simulink model "NHR9410Model96k_2020b"  (R2020b)
settings: Solver=ode45  StartTime=0.0  StopTime=1  FixedStep=0.001  MaxStep=20e-6  RelTol=1e-3
undefined symbols (not defined in the file): Ts
libraries: simulink x85, fl_lib x49, powerlib_meascontrol x27, simulink_extras x24, nesl_utility x13
(part 1 of 4)
settings Model: Creator=opal  LastModifiedBy=mne4
settings DataIOCC: ReturnWorkspaceOutputs=off
settings DebuggingCC: ParameterPrecisionLossMsg=none  ArithmeticOperatorsInVariantConditions=warning
settings SFSimCC: SimUseLocalCustomCode=off  CustomCodeUndefinedFunction=UseInterfaceOnly
settings RTWCC: RTWUseLocalCustomCode=off
settings CodeAppCC: StateflowObjectComments=on
settings SimscapeCC: SimscapeNormalizeSystem=off

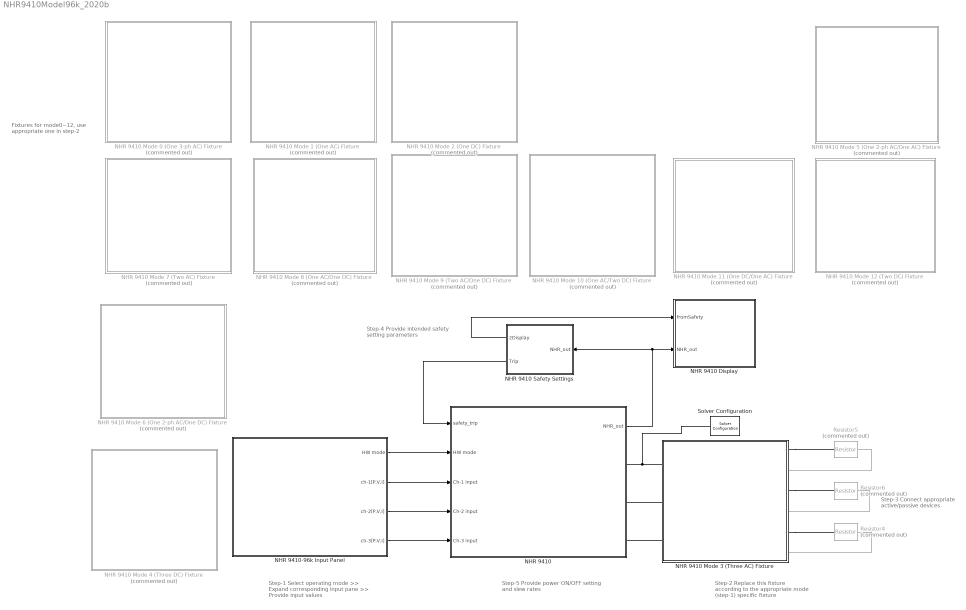
== system NHR9410Model96k_2020b ==
  note: Step-5
      | Provide power ON/OFF setting and slew rates
  note: Step-1
      | Select operating mode >> Expand corresponding input pane >> Provide input values
  note: Step-2
      | Replace this fixture according to the appropriate mode (step-1) specific fixture
  note: Step-3
      | Connect appropriate active/passive devices
  note: Step-4
      | Provide intended safety setting parameters
  note: Fixtures for mode0~12, use appropriate one in step-2
  NHR 9410 : Subsystem  mask{p_switch=1, VslewAC=0.0, FslewAC=500.0, VslewDC=0.0, IslewDC=0.0, PslewDC=0.0}
      mask prompts: p_switch "Enter 1 to turn ON, 0 to turn OFF NHR 9410"
      mask DialogControl DescTextVar Prompt: NHR 9410
      mask DialogControl Container3 Prompt: Slew Rates
      mask DialogControl Control2 Prompt: AC Voltage slew rate [0-500000V/s]:
      mask DialogControl f Prompt: Frequency slew rate [0-500 /s]
      mask DialogControl Control3 Prompt: DC Voltage slew rate [0-20000V/s]:
      mask DialogControl Control4 Prompt: DC current slew rate [0-100000A/s]:
      mask DialogControl Control5 Prompt: DC power slew rate [0-1000000W/s]:
      mask Display: image('NHR9410.png');
  NHR 9410 Display : Subsystem
  NHR 9410 Mode 0 (One 3-ph AC) Fixture : Subsystem  Commented=on
  NHR 9410 Mode 1 (One AC) Fixture : Subsystem  Commented=on
  NHR 9410 Mode 10 (One AC/Two DC) Fixture : Subsystem  Commented=on
  NHR 9410 Mode 11 (One DC/One AC) Fixture : Subsystem  Commented=on
  NHR 9410 Mode 12 (Two DC) Fixture : Subsystem  Commented=on
  NHR 9410 Mode 2 (One DC) Fixture : Subsystem  Commented=on
  NHR 9410 Mode 3 (Three AC) Fixture : Subsystem
  NHR 9410 Mode 4 (Three DC) Fixture : Subsystem  Commented=on
  NHR 9410 Mode 5 (One 2-ph AC/One AC) Fixture : Subsystem  Commented=on
  NHR 9410 Mode 6 (One 2-ph AC/One DC) Fixture : Subsystem  Commented=on
  NHR 9410 Mode 7 (Two AC) Fixture : Subsystem  Commented=on
  NHR 9410 Mode 8 (One AC/One DC) Fixture : Subsystem  Commented=on
  NHR 9410 Mode 9 (Two AC/One DC) Fixture : Subsystem  Commented=on
  NHR 9410 Safety Settings : Subsystem  mask{Vmin1=-50, Tvmin1=2, Svmin1=-1, Vmax1=100, Tvmax1=0.2, Svmax1=-1, Vpeak1=100, Vpeaken1=0, Imaxsrc1=80, Timaxsrc1=2, Simaxsrc1=-1, Imaxsnk1=50, Timaxsnk1=2, Simaxsnk1=-1, Ipeak1=80, Ipeaken1=0, Pmaxsrc1=2000, Tpmaxsrc1=2, Spmaxsrc1=-1, Pmaxsnk1=50, Tpmaxsnk1=2, Spmaxsnk1=-1, Vmin2=-50, Tvmin2=2, Svmin2=-1, Vmax2=90, Tvmax2=0.5, Svmax2=-1, Vpeak2=80, Vpeaken2=0, Imaxsrc2=50, Timaxsrc2=2, Simaxsrc2=-1, Imaxsnk2=8, Timaxsnk2=5, Simaxsnk2=1, Ipeak2=80, Ipeaken2=0, Pmaxsrc2=50, Tpmaxsrc2=2, Spmaxsrc2=-1, Pmaxsnk2=50, Tpmaxsnk2=2, Spmaxsnk2=-1, Vmin3=-50, Tvmin3=2, Svmin3=-1, Vmax3=500, Tvmax3=0.5, Svmax3=-1, Vpeak3=80, Vpeaken3=0, Imaxsrc3=50, Timaxsrc3=2, Simaxsrc3=-1, Imaxsnk3=8, Timaxsnk3=0.2, Simaxsnk3=-1, Ipeak3=80, Ipeaken3=0, Pmaxsrc3=50, Tpmaxsrc3=2, Spmaxsrc3=-1, Pmaxsnk3=3000, Tpmaxsnk3=0.2, Spmaxsnk3=1}
      mask prompts: Vmin1 "Min Voltage (V):"; Tvmin1 "Min Voltage time (S):"; Svmin1 "Enter (-1) to disable safety, 1 to enable:"; Vmax1 "Max Voltage (V):"; Tvmax1 "Max Voltage time (S):"; Svmax1 "Enter (-1) to disable safety, 1 to enable:"; Vpeak1 "Absolute Peak Voltage (V):"; Vpeaken1 "Enable Peak V Trip, yes/no (1/0):"; Imaxsrc1 "Max Source Current (A):"; Timaxsrc1 "Max Source Current Time (S):"; Simaxsrc1 "Enter (-1) to disable safety, 1 to enable:"; Imaxsnk1 "Max Sink Current (A):"; Timaxsnk1 "Max Sink Current Time (S):"; Simaxsnk1 "Enter (-1) to disable safety, 1 to enable:"; Ipeak1 "Absolute Peak Current (A):"; Ipeaken1 "Enable Peak A Trip, yes/no (1/0):"; Pmaxsrc1 "Max Source Power (W):"; Tpmaxsrc1 "Max Source Power Time (S):"; Spmaxsrc1 "Enter (-1) to disable safety, 1 to enable:"; Pmaxsnk1 "Max Sink Power (W):"; Tpmaxsnk1 "Max Sink Power Time (S):"; Spmaxsnk1 "Enter (-1) to disable safety, 1 to enable:"; Vmin2 "Min Voltage (V):"; Tvmin2 "Min Voltage time (S):"; Svmin2 "Enter (-1) to disable safety, 1 to enable:"; Vmax2 "Max Voltage (V):"; Tvmax2 "Max Voltage time (S):"; Svmax2 "Enter (-1) to disable safety, 1 to enable:"; Vpeak2 "Absolute Peak Voltage (V):"; Vpeaken2 "Enable Peak V Trip, yes/no (1/0):"; Imaxsrc2 "Max Source Current (A):"; Timaxsrc2 "Max Source Current Time (S):"; Simaxsrc2 "Enter (-1) to disable safety, 1 to enable:"; Imaxsnk2 "Max Sink Current (A):"; Timaxsnk2 "Max Sink Current Time (S):"; Simaxsnk2 "Enter (-1) to disable safety, 1 to enable:"; Ipeak2 "Absolute Peak Current (A):"; Ipeaken2 "Enable Peak A Trip, yes/no (1/0):"; Pmaxsrc2 "Max Source Power (W):"; Tpmaxsrc2 "Max Source Power Time (S):"; Spmaxsrc2 "Enter (-1) to disable safety, 1 to enable:"; Pmaxsnk2 "Max Sink Power (W):"; Tpmaxsnk2 "Max Sink Power Time (S):"; Spmaxsnk2 "Enter (-1) to disable safety, 1 to enable:"; Vmin3 "Min Voltage (V):"; Tvmin3 "Min Voltage time (S):"; Svmin3 "Enter (-1) to disable safety, 1 to enable:"; Vmax3 "Max Voltage (V):"; Tvmax3 "Max Voltage time (S):"; Svmax3 "Enter (-1) to disable safety, 1 to enable:"; Vpeak3 "Absolute Peak Voltage (V):"; Vpeaken3 "Enable Peak V Trip, yes/no (1/0):"; Imaxsrc3 "Max Source Current (A):"; Timaxsrc3 "Max Source Current Time (S):"; Simaxsrc3 "Enter (-1) to disable safety, 1 to enable:"; Imaxsnk3 "Max Sink Current (A):"; Timaxsnk3 "Max Sink Current Time (S):"; Simaxsnk3 "Enter (-1) to disable safety, 1 to enable:"; Ipeak3 "Absolute Peak Current (A):"; Ipeaken3 "Enable Peak A Trip, yes/no (1/0):"; Pmaxsrc3 "Max Source Power (W):"; Tpmaxsrc3 "Max Source Power Time (S):"; Spmaxsrc3 "Enter (-1) to disable safety, 1 to enable:"; Pmaxsnk3 "Max Sink Power (W):"; Tpmaxsnk3 "Max Sink Power Time (S):"; Spmaxsnk3 "Enter (-1) to disable safety, 1 to enable:"
      mask DialogControl DescTextVar Prompt: NHR 9410 Safety Settings
      mask DialogControl Container27 Prompt: Provide safety trip parameters
      mask DialogControl Container491 Prompt: Channel-1 safety trip settings
      mask DialogControl Container501 Prompt: Channel-2 safety trip settings
      mask DialogControl Container51 Prompt: Channel-3 safety trip settings
  NHR 9410-96k Input Panel : Subsystem  mask{sel=3, md0Pm1=80, md0Vrms1=277, md0Irms1=199.200, md0f1=60, md1Pm=96.0, md1Vrms=277, md1Irms=720.0, md1f=60, md1ph=0, md2Pm=96, md2Vm=400, md2Im=720, md3Pm1=20, md3Vrms1=277, md3Irms1=200, md3f1=60, md3ph1=0.0, md3Pm2=20, md3Vrms2=277, md3Irms2=200, md3f2=60, md3ph2=0, md3Pm3=20, md3Vrms3=277, md3Irms3=200, md3f3=60, md3ph3=0, md4Pm1=32, md4Vm1=400, md4Im1=232.800, md4Pm2=32.0, md4Vm2=400.0, md4Im2=240.0, md4Pm3=32.0, md4Vm3=400.0, md4Im3=240.0, md5Pm1=64.0, md5Vrms1=500, md5Irms1=240.0, md5f1=60, md5Pm2=32.0, md5Vrms2=350.0, md5Irms2=240.0, md5f2=60, md5ph2=0, md6Pm1=64, md6Vrms1=215.0, md6Irms1=240.0, md6f1=60, md6Pm2=32.0, md6Vm2=400.0, md6Im2=240.0, md7Pm1=64.0, md7Vrms1=277, md7Irms1=480.0, md7f1=60, md7ph1=0, md7Pm2=32.0, md7Vrms2=277, md7Irms2=240.0, md7f2=60, md7ph2=0, md8Pm1=32, md8Vrms1=277, md8Irms1=200, md8f1=60, md8ph1=0, md8Pm2=32, md8Vm2=400, md8Im2=200, md9Pm1=26.560, md9Vrms1=224.0, md9Irms1=240.0, md9f1=60, md9ph1=0, md9Pm2=32.0, md9Vrms2=277, md9Irms2=240.0, md9f2=60, md9ph2=0, md9Pm3=32.0, md9Vm3=400.0, md9Im3=240.0, md10Pm1=32.0, md10Vrms1=277, md10Irms1=237.600, md10f1=60, md10ph1=0, md10Pm2=2.240, md10Vm2=50, md10Im2=14.400, md10Pm3=31.680, md10Vm3=392.0, md10Im3=240.0, md11Pm1=64.0, md11Vm1=400.0, md11Im1=480.0, md11Pm2=32.0, md11Vrms2=277, md11Irms2=240.0, md11f2=60, md11ph2=0, md12Pm1=64, md12Vm1=400.0, md12Im1=480.0, md12Pm2=32.0, md12Vm2=400.0, md12Im2=240.0}
      mask prompts: sel "Enter corresponding index (0~12) for intended hardware operating mode selection:"
      mask DialogControl DescTextVar Prompt: NHR 9410-96k Input Panel
      mask DialogControl Container4 Prompt: 0: One 3-phase AC
      mask DialogControl Container66 Prompt: Expand to provide input parameters
      mask DialogControl Container47 Prompt: General operating input
      mask DialogControl Control2 Prompt: Maximum power (kW) [0-96kW]:
      mask DialogControl Control3 Prompt: Maximum voltage (Vrms l-n) [0-350V]:
      mask DialogControl Control4 Prompt: Maximum current per phase (Arms) [0-240A]:
      mask DialogControl Control5 Prompt: Frequency (Hz) [30-100Hz]:
      mask DialogControl Control6 Prompt: Phase angle (degrees) [phase-A]: 0
      mask DialogControl Control7 Prompt: Phase angle (degrees) [phase-B]: 240
      mask DialogControl Control8 Prompt: Phase angle (degrees) [phase-C]: 120
      mask DialogControl Container21 Prompt: 1: One AC
      mask DialogControl Container74 Prompt: Expand to provide input parameters
      mask DialogControl Control30 Prompt: Maximum power (kW) [0-96kW]:
      mask DialogControl Control31 Prompt: Maximum voltage (Vrms l-n) [0-350V]:
      mask DialogControl Control32 Prompt: Maximum current (Arms) [0-720A]:
      mask DialogControl Control33 Prompt: Frequency (Hz) [30-100Hz]:
      mask DialogControl Control34 Prompt: Phase angle (degrees):
      mask DialogControl Container24 Prompt: 2: One DC
      mask DialogControl Container76 Prompt: Expand to provide input parameters
      mask DialogControl Control18 Prompt: Maximum power (kW) [0-96kW]:
      mask DialogControl Control19 Prompt: Maximum voltage (Vdc) [0-400V]:
      mask DialogControl Control20 Prompt: Maximum current (A) [0-720A]:
      mask DialogControl Container27 Prompt: 3: Three AC
      mask DialogControl Container78 Prompt: Expand to provide input parameters
      mask DialogControl Container104 Prompt: AC-1 (chanel-1) input
      mask DialogControl Control40 Prompt: Maximum power (kW) [0-32kW]:
      mask DialogControl Control41 Prompt: Maximum voltage (Vrms l-n) [0-350V]:
      mask DialogControl Control42 Prompt: Maximum current (Arms) [0-240A]:
      mask DialogControl Control43 Prompt: Frequency (Hz) [30-100Hz]:
      mask DialogControl Control44 Prompt: Phase angle (degrees):
      mask DialogControl Container105 Prompt: AC-2 (chanel-2) input
      mask DialogControl Control45 Prompt: Maximum power (kW) [0-32kW]:
      mask DialogControl Control46 Prompt: Maximum voltage (Vrms l-n) [0-350V]:
      mask DialogControl Control47 Prompt: Maximum current (Arms) [0-240A]:
      mask DialogControl Control48 Prompt: Frequency (Hz) [30-100Hz]:
      mask DialogControl Control49 Prompt: Phase angle (degrees):
      mask DialogControl Control50 Prompt: Maximum power (kW) [0-32kW]:
      mask DialogControl Control51 Prompt: Maximum voltage (Vrms l-n) [0-350V]:
      mask DialogControl Control52 Prompt: Maximum current (Arms) [0-240A]:
      mask DialogControl Control53 Prompt: Frequency (Hz) [30-100Hz]:
      mask DialogControl Control54 Prompt: Phase angle (degrees):
      mask DialogControl Container30 Prompt: 4: Three DC
      mask DialogControl Container71 Prompt: Expand to provide input parameters
      mask DialogControl Container58 Prompt: Chanel-1 input
      mask DialogControl Control9 Prompt: Maximum power (kW) [0-32kW]:
      mask DialogControl Control10 Prompt: Maximum voltage (Vdc) [0-400V]:
      mask DialogControl Control11 Prompt: Mximum current (A) [0-240A]:
      mask DialogControl Container63 Prompt: Chanel-2 input
      mask DialogControl Control12 Prompt: Maximum power (kW) [0-32kW]:
      mask DialogControl Control13 Prompt: Maximum voltage (Vdc) [0-400V]:
      mask DialogControl Control14 Prompt: Maximum current (A) [0-240A]:
      mask DialogControl Container65 Prompt: Chanel-3 input
      mask DialogControl Control15 Prompt: Maximum power (kW) [0-32kW]:
      mask DialogControl Control16 Prompt: Maximum voltage (Vdc) [0-400V]:
      mask DialogControl Control17 Prompt: Maximum current (A) [0-240A]:
      mask DialogControl Container33 Prompt: 5: One 2-ph AC and one AC
      mask DialogControl Container80 Prompt: Expand to provide input parameters
      mask DialogControl Container127 Prompt: AC-1 (2-ph) (chanel 1,2) Input
      mask DialogControl Control152 Prompt: Maximum power (kW) [0-64kW]:
      mask DialogControl Control153 Prompt: Maximum voltage (Vrms l-l) [0-500V]:
      mask DialogControl Control154 Prompt: Maximum current per phase (Arms) [0-240A]:
      mask DialogControl Control155 Prompt: Frequency (Hz) [30-100Hz]:
      mask DialogControl Control161 Prompt: Phase angle (degrees): A=0, B=180
      mask DialogControl Container128 Prompt: AC-3 (chanel 3) Input
      mask DialogControl Control156 Prompt: Maximum power (kW) [0-32kW]:
      mask DialogControl Control157 Prompt: Maximum voltage (Vrms l-n) [0-350V]:
      mask DialogControl Control158 Prompt: Maximum current (Arms) [0-240A]:
      mask DialogControl Control159 Prompt: Frequency (Hz) [30-100Hz]:
      mask DialogControl Control160 Prompt: Phase angle (degrees):
      mask DialogControl Container36 Prompt: 6: One 2-ph AC and one DC
      mask DialogControl Container82 Prompt: Expand to provide input parameters
      mask DialogControl Container131 Prompt: AC-1 (2-ph) (chanel 1,2) Input
      mask DialogControl Control162 Prompt: Maximum power (kW) [0-64kW]:
      mask DialogControl Control163 Prompt: Maximum voltage (Vrms l-l) [0-500V]:
      mask DialogControl Control164 Prompt: Maximum current per phase (Arms) [0-240A]:
      mask DialogControl Control165 Prompt: Frequency (Hz) [30-100Hz]:
      mask DialogControl Control169 Prompt: Phase angle (degrees): A=0, B=180
      mask DialogControl Container132 Prompt: DC-3 (chanel 3) Input
      mask DialogControl Control166 Prompt: Maximum power (kW) [0-32kW]:
      mask DialogControl Control167 Prompt: Maximum voltage (Vdc) [0-400V]:
      mask DialogControl Control168 Prompt: Maximum current (A) [0-240A]:
      mask DialogControl Container39 Prompt: 7: Two AC
      mask DialogControl Container84 Prompt: Expand to provide input parameters
      mask DialogControl Container107 Prompt: AC-1 (chanel 1,2) input
      mask DialogControl Control70 Prompt: Maximum power (kW) [0-64kW]:
      mask DialogControl Control71 Prompt: Maximum voltage (Vrms l-n) [0-350V]:
      mask DialogControl Control72 Prompt: Maximum current (Arms) [0-480A]:
      mask DialogControl Control73 Prompt: Frequency (Hz) [30-100Hz]:
      mask DialogControl Control74 Prompt: Phase angle (degrees):
      mask DialogControl Container108 Prompt: AC-3 (chanel 3)input
      mask DialogControl Control75 Prompt: Maximum power (kW) [0-32kW]:
      mask DialogControl Control76 Prompt: Maximum voltage (Vrms l-n) [0-350V]:
      mask DialogControl Control77 Prompt: Maximum current (Arms) [0-240A]:
      mask DialogControl Control78 Prompt: Frequency (Hz) [30-100Hz]:
      mask DialogControl Control79 Prompt: Phase angle (degrees):
      mask DialogControl Container42 Prompt: 8: One AC and one DC
      mask DialogControl Container86 Prompt: Expand to provide input parameters
      mask DialogControl Container110 Prompt: AC-1 (chanel 1,2) input
      mask DialogControl Control86 Prompt: Maximum power (kW) [0-64kW]:
      mask DialogControl Control87 Prompt: Maximum voltage (Vrms l-n) [0-350V]:
      mask DialogControl Control88 Prompt: Maximum current (Arms) [0-480A]:
      mask DialogControl Control89 Prompt: Frequency (Hz) [30-100Hz]:
      mask DialogControl Control90 Prompt: Phase angle (degrees):
      mask DialogControl Container111 Prompt: DC-3 (chanel 3) input
      mask DialogControl Control91 Prompt: Maximum power (kW) [0-32kW]:
      mask DialogControl Control92 Prompt: Maximum voltage (Vdc) [0-400V]:
      mask DialogControl Control93 Prompt: Maximum current (A) [0-240A]:
      mask DialogControl Container49 Prompt: 9: Two AC and One DC
      mask DialogControl Container88 Prompt: Expand to provide input parameters
      mask DialogControl Container123 Prompt: AC-1 (chanel 1) input
      mask DialogControl Control130 Prompt: Maximum power (kW) [0-32kW]:
      mask DialogControl Control131 Prompt: Maximum voltage (Vrms l-n) [0-350V]:
      mask DialogControl Control132 Prompt: Maximum current (Arms) [0-240A]:
      mask DialogControl Control133 Prompt: Frequency (Hz) [30-100Hz]:
      mask DialogControl Control134 Prompt: Phase angle (degrees):
      mask DialogControl Container125 Prompt: AC-2 (chanel 2) input
      mask DialogControl Control135 Prompt: Maximum power (kW) [0-32kW]:
      mask DialogControl Control136 Prompt: Maximum voltage (Vrms l-n) [0-350V]:
      mask DialogControl Control137 Prompt: Maximum current (Arms) [0-240A]:
      mask DialogControl Control138 Prompt: Frequency (Hz) [30-100Hz]:
      mask DialogControl Control139 Prompt: Phase angle (degrees):
      mask DialogControl Container126 Prompt: DC-3 (chanel 3) input
      mask DialogControl Control140 Prompt: Maximum power (kW) [0-32kW]:
      mask DialogControl Control141 Prompt: Maximum voltage (Vdc) [0-400V]:
      mask DialogControl Control142 Prompt: Maximum current (A) [0-240A]:
      mask DialogControl Container52 Prompt: 10: One AC and Two DC
      mask DialogControl Container90 Prompt: Expand to provide input parameters
      mask DialogControl Container117 Prompt: AC-1 (chanel 1) input
      mask DialogControl Control114 Prompt: Maximum power (kW) [0-32kW]:
      mask DialogControl Control115 Prompt: Maximum voltage (Vrms l-n) [0-350V]:
      mask DialogControl Control116 Prompt: Maximum current (Arms) [0-240A]:
      mask DialogControl Control117 Prompt: Frequency (Hz) [30-100Hz]:
      mask DialogControl Control118 Prompt: Phase angle (degrees):
      mask DialogControl Container118 Prompt: DC-2 (chanel 2) input
      mask DialogControl Control119 Prompt: Maximum power (kW) [0-32kW]:
      mask DialogControl Control120 Prompt: Maximum voltage (Vdc) [0-400V]:
      mask DialogControl Control121 Prompt: Maximum current (A) [0-240A]:
      mask DialogControl Container119 Prompt: DC-3 (chanel 3) input
      mask DialogControl Control122 Prompt: Maximum power (kW) [0-32kW]:
      mask DialogControl Control123 Prompt: Maximum voltage (Vdc) [0-400V]:
      mask DialogControl Control124 Prompt: Maximum current (A) [0-240A]:
      mask DialogControl Container60 Prompt: 11: One DC and One AC
      mask DialogControl Container92 Prompt: Expand to provide input parameters
      mask DialogControl Container113 Prompt: DC-1 (chanel 1,2) input
      mask DialogControl Control100 Prompt: Maximum power (kW) [0-64kW]:
      mask DialogControl Control101 Prompt: Maximum voltage (Vdc) [0-400V]:
      mask DialogControl Control102 Prompt: Maximum current (A) [0-480A]:
      mask DialogControl Container114 Prompt: AC-3 (chanel 3) input
      mask DialogControl Control103 Prompt: Maximum power (kW) [0-32kW]:
      mask DialogControl Control104 Prompt: Maximum voltage (Vrms l-n) [0-350V]:
      mask DialogControl Control105 Prompt: Maximum current (Arms) [0-240A]:
      mask DialogControl Control106 Prompt: Frequency (Hz) [30-100Hz]:
      mask DialogControl Control107 Prompt: Phase angle (degrees):
      mask DialogControl Container68 Prompt: 12: Two DC
      mask DialogControl Container94 Prompt: Expand to provide input parameters
      mask DialogControl Container100 Prompt: DC-1 (chanel 1,2) input
      mask DialogControl Control24 Prompt: Maximum power (kW) [0-64kW]:
      mask DialogControl Control25 Prompt: Maximum voltage (Vdc) [0-400V]:
      mask DialogControl Control26 Prompt: Maximum current (A) [0-480A]:
      mask DialogControl Container102 Prompt: DC-3 (chanel 3) input
      mask DialogControl Control27 Prompt: Maximum power (kW) [0-32kW]:
      mask DialogControl Control28 Prompt: Maximum voltage (Vdc) [0-400V]:
      mask DialogControl Control29 Prompt: Maximum current (A) [0-240A]:
      mask Display: image('NHR9410Model96k.png');
  Resistor4 : fl_lib/Electrical/Electrical Elements/Resistor  Commented=on  R=1.66 Ohm  i_specify=off  i_priority=None  i=0 A  i_nominal_specify=off  i_nominal_unit=A  i_nominal_value=1  v_specify=off  v_priority=None  v=0 V  v_nominal_specify=off  v_nominal_unit=V  v_nominal_value=1
  Resistor5 : fl_lib/Electrical/Electrical Elements/Resistor  Commented=on  R=1.66 Ohm  i_specify=off  i_priority=None  i=0 A  i_nominal_specify=off  i_nominal_unit=A  i_nominal_value=1  v_specify=off  v_priority=None  v=0 V  v_nominal_specify=off  v_nominal_unit=V  v_nominal_value=1
  Resistor6 : fl_lib/Electrical/Electrical Elements/Resistor  Commented=on  R=1.66 Ohm  i_specify=off  i_priority=None  i=0 A  i_nominal_specify=off  i_nominal_unit=A  i_nominal_value=1  v_specify=off  v_priority=None  v=0 V  v_nominal_specify=off  v_nominal_unit=V  v_nominal_value=1
  Solver Configuration : nesl_utility/Solver Configuration  PhysicalDomain=network_engine_domain  SubClassName=solver  LeftPortType=input  RightPortType=generic  Tones=[]  Harmonics=[]  SimulateNoise=off  Profile=off  UseLocalSampling=off  EnableSwitchedLinearOptims=on  FrequencyDomain=off  UseCCode=off  RelTol=0.001  AbsTol=1e-06  MinStep=1e-09  ToWorkspace=off  RevertToSquareIcSolve=off  NumHomotopyIterations=100  PhasorMode=off  PhasorModeNumHarmonics=1  DoDC=on  ResidualTolerance=1e-09  UseLocalSolver=on  LocalSolverChoice=NE_BACKWARD_EULER_ADVANCER  LocalSolverSampleTime=0.001  DoFixedCost=on  MaxNonlinIter=3  MaxModeIter=2  ComputeImpulses=off  ImpulseIterations=2  LinearAlgebra=Sparse  EquationFormulation=NE_TIME_EF  DelaysMemoryBudget=1024  AutomaticFiltering=off  FilteringTimeConstant=0.001  PartitionStorageMethod=AS_NEEDED  PartitionMemoryBudget=1024  PartitionMethod=FAST
  wires:
  NHR 9410-96k Input Panel/1(HW mode) -> NHR 9410/2(HW mode)
  NHR 9410-96k Input Panel/2(ch-1[P,V,I]) -> NHR 9410/3(Ch-1 input)
  NHR 9410-96k Input Panel/3(ch-2[P,V,I]) -> NHR 9410/4(Ch-2 input)
  NHR 9410-96k Input Panel/4(ch-3[P,V,I]) -> NHR 9410/5(Ch-3 input)
  NHR 9410/1(NHR_out) -> NHR 9410 Safety Settings/1(NHR_out), NHR 9410 Display/2(NHR_out)
  NHR 9410 Safety Settings/2(Trip) -> NHR 9410/1(safety_trip)
  NHR 9410 Safety Settings/1(2Display) -> NHR 9410 Display/1(fromSafety)
  connections:
  NHR 9410 Mode 3 (Three AC) Fixture/LConn1 -- Solver Configuration/RConn1 -- NHR 9410/RConn1
  NHR 9410 Mode 3 (Three AC) Fixture/LConn2 -- NHR 9410/RConn2
  NHR 9410 Mode 3 (Three AC) Fixture/LConn3 -- NHR 9410/RConn3
  NHR 9410 Mode 3 (Three AC) Fixture/RConn1 -- Resistor5/LConn1
  NHR 9410 Mode 3 (Three AC) Fixture/RConn3 -- Resistor6/LConn1
  NHR 9410 Mode 3 (Three AC) Fixture/RConn5 -- Resistor4/LConn1
  Resistor5/RConn1 -- NHR 9410 Mode 3 (Three AC) Fixture/RConn2
  Resistor6/RConn1 -- NHR 9410 Mode 3 (Three AC) Fixture/RConn4
  Resistor4/RConn1 -- NHR 9410 Mode 3 (Three AC) Fixture/RConn6

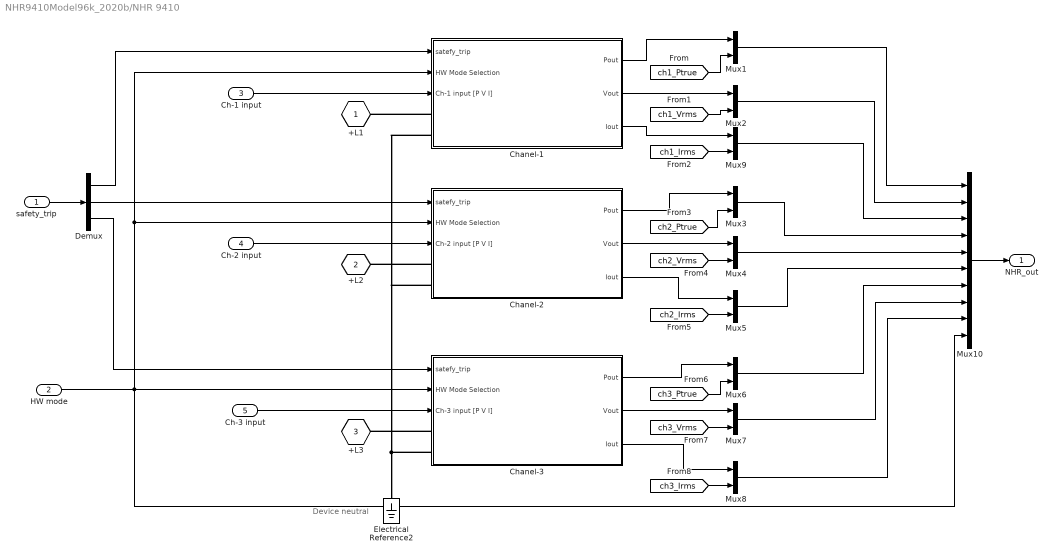
== system NHR9410Model96k_2020b/NHR 9410 ==
  note: Device neutral
  safety_trip : Inport
  HW mode : Inport  Port=2
  Ch-1 input : Inport  Port=3
  Ch-2 input : Inport  Port=4
  Ch-3 input : Inport  Port=5
  Chanel-1 : Subsystem
  Chanel-2 : Subsystem
  Chanel-3 : Subsystem
  Demux : Demux  Outputs=3
  Electrical Reference2 : fl_lib/Electrical/Electrical Elements/Electrical Reference
  Mux{1..9} (9 alike) : Mux  Inputs=2
  Mux10 : Mux  Inputs=10
  +L1 : PMIOPort  Side=Right
  +L2 : PMIOPort  Port=2  Side=Right
  +L3 : PMIOPort  Port=3  Side=Right
  NHR_out : Outport  VectorParamsAs1DForOutWhenUnconnected=off
  wires:
  Ch-3 input/1 -> Chanel-3/3(Ch-3 input [P V I])
  Ch-1 input/1 -> Chanel-1/3(Ch-1 input [P V I])
  Ch-2 input/1 -> Chanel-2/3(Ch-2 input [P V I])
  Chanel-2/1(Pout) -> Mux3/1
  Chanel-2/2(Vout) -> Mux4/1
  Chanel-2/3(Iout) -> Mux5/1
  Chanel-3/1(Pout) -> Mux6/1
  Chanel-3/2(Vout) -> Mux7/1
  Chanel-3/3(Iout) -> Mux8/1
  [ch2_Ptrue] -> Mux3/2
  [ch2_Vrms] -> Mux4/2
  [ch2_Irms] -> Mux5/2
  [ch3_Ptrue] -> Mux6/2
  [ch3_Vrms] -> Mux7/2
  [ch3_Irms] -> Mux8/2
  Mux1/1 -> Mux10/1
  Mux2/1 -> Mux10/2
  Mux9/1 -> Mux10/3
  Mux3/1 -> Mux10/4
  Mux4/1 -> Mux10/5
  Mux6/1 -> Mux10/7
  Mux7/1 -> Mux10/8
  Mux8/1 -> Mux10/9
  Demux/2 -> Chanel-2/1(satefy_trip)
  Demux/1 -> Chanel-1/1(satefy_trip)
  safety_trip/1 -> Demux/1
  Demux/3 -> Chanel-3/1(satefy_trip)
  Mux5/1 -> Mux10/6
  HW mode/1 -> Chanel-2/2(HW Mode Selection), Chanel-1/2(HW Mode Selection), Mux10/10, Chanel-3/2(HW Mode Selection)
  Mux10/1 -> NHR_out/1
  Chanel-1/2(Vout) -> Mux2/1
  Chanel-1/1(Pout) -> Mux1/1
  Chanel-1/3(Iout) -> Mux9/1
  [ch1_Ptrue] -> Mux1/2
  [ch1_Vrms] -> Mux2/2
  [ch1_Irms] -> Mux9/2
  connections:
  Chanel-1/LConn1 -- +L1/RConn1
  Chanel-2/LConn1 -- +L2/RConn1
  Chanel-3/LConn1 -- +L3/RConn1
  Chanel-3/LConn2 -- Chanel-1/LConn2 -- Chanel-2/LConn2 -- Electrical Reference2/LConn1

== system NHR9410Model96k_2020b/NHR 9410 Display ==
  note: ch-3 I/Irms
  note: ch-3 V/Vrms
  note: ch-3 P/Ptrue
  note: ch-2 I/Irms
  note: ch-2 V/Vrms
  note: ch-2 P/Ptrue
  note: ch-1 I/Irms
  note: ch-1 V/Vrms
  note: ch-1 P/Ptrue
  note: Pmax(snk)
  note: Pmax(src)
  note: Ipeak
  note: Imax(snk)
  note: Imax(src)
  note: Vpeak
  note: Vmax
  note: Vmin
  note: ch-1
  note: Pmax(snk)
  note: Pmax(src)
  note: Ipeak
  note: Imax(snk)
  note: Imax(src)
  note: Vpeak
  note: Vmax
  note: Vmin
  note: ch-2
  note: Pmax(snk)
  note: Pmax(src)
  note: Ipeak
  note: Imax(snk)
  note: Imax(src)
  note: Vpeak
  note: Vmax
  note: Vmin
  note: ch-3
  fromSafety : Inport
  NHR_out : Inport  Port=2
  Ch-1 all safety : Scope  NumInputPorts=9
  Ch-2 all safety : Scope  NumInputPorts=9
  Ch-3 all safety : Scope  NumInputPorts=9
  Chanel-[1,2,3] [P V I] : Scope  NumInputPorts=9
  Demux : Demux  Outputs=10
  Demux1 : Demux  Outputs=3
  Demux2 : Demux  Outputs=9
  Demux3 : Demux  Outputs=9
  Demux4 : Demux  Outputs=9
  Scope : Scope  NumInputPorts=3
  op_mode : Display
  wires:
  Demux/6 -> Chanel-[1,2,3] [P V I]/6
  Demux/9 -> Chanel-[1,2,3] [P V I]/9
  Demux/3 -> Chanel-[1,2,3] [P V I]/3
  Demux/8 -> Chanel-[1,2,3] [P V I]/8
  Demux/5 -> Chanel-[1,2,3] [P V I]/5
  Demux/2 -> Chanel-[1,2,3] [P V I]/2
  NHR_out/1 -> Demux/1
  Demux/4 -> Chanel-[1,2,3] [P V I]/4
  Demux/1 -> Chanel-[1,2,3] [P V I]/1
  Demux/7 -> Chanel-[1,2,3] [P V I]/7
  Demux/10 -> op_mode/1
  fromSafety/1 -> Demux1/1
  Demux1/1 -> Demux2/1
  Demux1/2 -> Demux3/1
  Demux1/3 -> Demux4/1
  Demux2/1 -> Scope/1, Ch-1 all safety/1
  Demux2/9 -> Ch-1 all safety/9
  Demux2/8 -> Ch-1 all safety/8
  Demux2/7 -> Ch-1 all safety/7
  Demux2/6 -> Ch-1 all safety/6
  Demux2/5 -> Ch-1 all safety/5
  Demux2/4 -> Ch-1 all safety/4
  Demux2/3 -> Ch-1 all safety/3
  Demux2/2 -> Ch-1 all safety/2
  Demux3/2 -> Ch-2 all safety/2
  Demux3/3 -> Ch-2 all safety/3
  Demux3/4 -> Ch-2 all safety/4
  Demux3/5 -> Ch-2 all safety/5
  Demux3/6 -> Ch-2 all safety/6
  Demux3/7 -> Ch-2 all safety/7
  Demux3/8 -> Ch-2 all safety/8
  Demux3/9 -> Ch-2 all safety/9
  Demux3/1 -> Scope/2, Ch-2 all safety/1
  Demux4/1 -> Scope/3, Ch-3 all safety/1
  Demux4/9 -> Ch-3 all safety/9
  Demux4/8 -> Ch-3 all safety/8
  Demux4/7 -> Ch-3 all safety/7
  Demux4/6 -> Ch-3 all safety/6
  Demux4/5 -> Ch-3 all safety/5
  Demux4/4 -> Ch-3 all safety/4
  Demux4/3 -> Ch-3 all safety/3
  Demux4/2 -> Ch-3 all safety/2

== system NHR9410Model96k_2020b/NHR 9410 Mode 0 (One 3-ph AC) Fixture ==
  note: Channel neutral
  Electrical Reference1 : fl_lib/Electrical/Electrical Elements/Electrical Reference
  +L1 : PMIOPort  Side=Left
  +L2 : PMIOPort  Port=2  Side=Left
  +L3 : PMIOPort  Port=3  Side=Left
  ph-A : PMIOPort  Port=4  Side=Right
  ph-B : PMIOPort  Port=5  Side=Right
  ph-C : PMIOPort  Port=6  Side=Right
  N : PMIOPort  Port=7  Side=Right
  connections:
  ph-A/RConn1 -- +L1/RConn1
  Electrical Reference1/LConn1 -- N/RConn1
  +L3/RConn1 -- ph-C/RConn1
  +L2/RConn1 -- ph-B/RConn1

== system NHR9410Model96k_2020b/NHR 9410 Mode 1 (One AC) Fixture ==
  note: Channel neutral
  Electrical Reference1 : fl_lib/Electrical/Electrical Elements/Electrical Reference
  +L1 : PMIOPort  Side=Left
  +L2 : PMIOPort  Port=2  Side=Left
  +L3 : PMIOPort  Port=3  Side=Left
  L : PMIOPort  Port=4  Side=Right
  N : PMIOPort  Port=5  Side=Right
  connections:
  Electrical Reference1/LConn1 -- N/RConn1
  L/RConn1 -- +L1/RConn1

== system NHR9410Model96k_2020b/NHR 9410 Mode 10 (One AC//Two DC) Fixture ==
  note: Channel neutral
  Electrical Reference1 : fl_lib/Electrical/Electrical Elements/Electrical Reference
  Electrical Reference2 : fl_lib/Electrical/Electrical Elements/Electrical Reference
  Electrical Reference3 : fl_lib/Electrical/Electrical Elements/Electrical Reference
  +L1 : PMIOPort  Side=Left
  +L2 : PMIOPort  Port=2  Side=Left
  +L3 : PMIOPort  Port=3  Side=Left
  L : PMIOPort  Port=4  Side=Right
  N : PMIOPort  Port=5  Side=Right
  V1+ : PMIOPort  Port=6  Side=Right
  V1- : PMIOPort  Port=7  Side=Right
  V2+ : PMIOPort  Port=8  Side=Right
  V2- : PMIOPort  Port=9  Side=Right
  connections:
  Electrical Reference1/LConn1 -- N/RConn1
  L/RConn1 -- +L1/RConn1
  Electrical Reference2/LConn1 -- V1-/RConn1
  Electrical Reference3/LConn1 -- V2-/RConn1
  +L2/RConn1 -- V1+/RConn1
  +L3/RConn1 -- V2+/RConn1

== system NHR9410Model96k_2020b/NHR 9410 Mode 11 (One DC//One AC) Fixture ==
  note: Channel neutral
  Electrical Reference1 : fl_lib/Electrical/Electrical Elements/Electrical Reference
  Electrical Reference3 : fl_lib/Electrical/Electrical Elements/Electrical Reference
  +L1 : PMIOPort  Side=Left
  +L2 : PMIOPort  Port=2  Side=Left
  +L3 : PMIOPort  Port=3  Side=Left
  V+ : PMIOPort  Port=4  Side=Right
  V- : PMIOPort  Port=5  Side=Right
  L : PMIOPort  Port=6  Side=Right
  N : PMIOPort  Port=7  Side=Right
  connections:
  Electrical Reference1/LConn1 -- V-/RConn1
  V+/RConn1 -- +L1/RConn1
  Electrical Reference3/LConn1 -- N/RConn1
  +L3/RConn1 -- L/RConn1

== system NHR9410Model96k_2020b/NHR 9410 Mode 12 (Two DC) Fixture ==
  note: Channel neutral
  Electrical Reference1 : fl_lib/Electrical/Electrical Elements/Electrical Reference
  Electrical Reference3 : fl_lib/Electrical/Electrical Elements/Electrical Reference
  +L1 : PMIOPort  Side=Left
  +L2 : PMIOPort  Port=2  Side=Left
  +L3 : PMIOPort  Port=3  Side=Left
  V1+ : PMIOPort  Port=4  Side=Right
  V1- : PMIOPort  Port=5  Side=Right
  V2+ : PMIOPort  Port=6  Side=Right
  V2- : PMIOPort  Port=7  Side=Right
  connections:
  +L3/RConn1 -- V2+/RConn1
  Electrical Reference3/LConn1 -- V2-/RConn1
  V1+/RConn1 -- +L1/RConn1
  Electrical Reference1/LConn1 -- V1-/RConn1

== system NHR9410Model96k_2020b/NHR 9410 Mode 2 (One DC) Fixture ==
  note: Channel neutral
  Electrical Reference1 : fl_lib/Electrical/Electrical Elements/Electrical Reference
  +L1 : PMIOPort  Side=Left
  +L2 : PMIOPort  Port=2  Side=Left
  +L3 : PMIOPort  Port=3  Side=Left
  V+ : PMIOPort  Port=4  Side=Right
  V- : PMIOPort  Port=5  Side=Right
  connections:
  V+/RConn1 -- +L1/RConn1
  Electrical Reference1/LConn1 -- V-/RConn1

== system NHR9410Model96k_2020b/NHR 9410 Mode 3 (Three AC) Fixture ==
  note: Channel neutral
  Electrical Reference1 : fl_lib/Electrical/Electrical Elements/Electrical Reference
  Electrical Reference2 : fl_lib/Electrical/Electrical Elements/Electrical Reference
  Electrical Reference3 : fl_lib/Electrical/Electrical Elements/Electrical Reference
  +L1 : PMIOPort  Side=Left
  +L2 : PMIOPort  Port=2  Side=Left
  +L3 : PMIOPort  Port=3  Side=Left
  L1 : PMIOPort  Port=4  Side=Right
  N1 : PMIOPort  Port=5  Side=Right
  L2 : PMIOPort  Port=6  Side=Right
  N2 : PMIOPort  Port=7  Side=Right
  L3 : PMIOPort  Port=8  Side=Right
  N3 : PMIOPort  Port=9  Side=Right
  connections:
  Electrical Reference1/LConn1 -- N1/RConn1
  L1/RConn1 -- +L1/RConn1
  Electrical Reference2/LConn1 -- N2/RConn1
  Electrical Reference3/LConn1 -- N3/RConn1
  +L2/RConn1 -- L2/RConn1
  +L3/RConn1 -- L3/RConn1

== system NHR9410Model96k_2020b/NHR 9410 Mode 4 (Three DC) Fixture ==
  note: Channel neutral
  Electrical Reference1 : fl_lib/Electrical/Electrical Elements/Electrical Reference
  Electrical Reference2 : fl_lib/Electrical/Electrical Elements/Electrical Reference
  Electrical Reference3 : fl_lib/Electrical/Electrical Elements/Electrical Reference
  +L1 : PMIOPort  Side=Left
  +L2 : PMIOPort  Port=2  Side=Left
  +L3 : PMIOPort  Port=3  Side=Left
  V1+ : PMIOPort  Port=4  Side=Right
  V1- : PMIOPort  Port=5  Side=Right
  V2+ : PMIOPort  Port=6  Side=Right
  V2- : PMIOPort  Port=7  Side=Right
  V3+ : PMIOPort  Port=8  Side=Right
  V3- : PMIOPort  Port=9  Side=Right
  connections:
  +L3/RConn1 -- V3+/RConn1
  +L2/RConn1 -- V2+/RConn1
  Electrical Reference3/LConn1 -- V3-/RConn1
  Electrical Reference2/LConn1 -- V2-/RConn1
  V1+/RConn1 -- +L1/RConn1
  Electrical Reference1/LConn1 -- V1-/RConn1

== system NHR9410Model96k_2020b/NHR 9410 Mode 5 (One 2-ph AC//One AC) Fixture ==
  note: Channel neutral
  Electrical Reference1 : fl_lib/Electrical/Electrical Elements/Electrical Reference
  Electrical Reference3 : fl_lib/Electrical/Electrical Elements/Electrical Reference
  +L1 : PMIOPort  Side=Left
  +L2 : PMIOPort  Port=2  Side=Left
  +L3 : PMIOPort  Port=3  Side=Left
  ph-A : PMIOPort  Port=4  Side=Right
  ph-B : PMIOPort  Port=5  Side=Right
  Nab : PMIOPort  Port=6  Side=Right
  L : PMIOPort  Port=7  Side=Right
  N : PMIOPort  Port=8  Side=Right
  connections:
  Electrical Reference1/LConn1 -- Nab/RConn1
  ph-A/RConn1 -- +L1/RConn1
  Electrical Reference3/LConn1 -- N/RConn1
  +L2/RConn1 -- ph-B/RConn1
  +L3/RConn1 -- L/RConn1

== system NHR9410Model96k_2020b/NHR 9410 Mode 6 (One 2-ph AC//One DC) Fixture ==
  note: Channel neutral
  Electrical Reference1 : fl_lib/Electrical/Electrical Elements/Electrical Reference
  Electrical Reference3 : fl_lib/Electrical/Electrical Elements/Electrical Reference
  +L1 : PMIOPort  Side=Left
  +L2 : PMIOPort  Port=2  Side=Left
  +L3 : PMIOPort  Port=3  Side=Left
  ph-A : PMIOPort  Port=4  Side=Right
  ph-B : PMIOPort  Port=5  Side=Right
  Nab : PMIOPort  Port=6  Side=Right
  V+ : PMIOPort  Port=7  Side=Right
  V- : PMIOPort  Port=8  Side=Right
  connections:
  +L3/RConn1 -- V+/RConn1
  +L2/RConn1 -- ph-B/RConn1
  Electrical Reference3/LConn1 -- V-/RConn1
  ph-A/RConn1 -- +L1/RConn1
  Electrical Reference1/LConn1 -- Nab/RConn1

== system NHR9410Model96k_2020b/NHR 9410 Mode 7 (Two AC) Fixture ==
  note: Channel neutral
  Electrical Reference1 : fl_lib/Electrical/Electrical Elements/Electrical Reference
  Electrical Reference3 : fl_lib/Electrical/Electrical Elements/Electrical Reference
  +L1 : PMIOPort  Side=Left
  +L2 : PMIOPort  Port=2  Side=Left
  +L3 : PMIOPort  Port=3  Side=Left
  L1 : PMIOPort  Port=4  Side=Right
  N1 : PMIOPort  Port=5  Side=Right
  L2 : PMIOPort  Port=6  Side=Right
  N2 : PMIOPort  Port=7  Side=Right
  connections:
  Electrical Reference1/LConn1 -- N1/RConn1
  L1/RConn1 -- +L1/RConn1
  Electrical Reference3/LConn1 -- N2/RConn1
  +L3/RConn1 -- L2/RConn1

== system NHR9410Model96k_2020b/NHR 9410 Mode 8 (One AC//One DC) Fixture ==
  note: Channel neutral
  Electrical Reference1 : fl_lib/Electrical/Electrical Elements/Electrical Reference
  Electrical Reference3 : fl_lib/Electrical/Electrical Elements/Electrical Reference
  +L1 : PMIOPort  Side=Left
  +L2 : PMIOPort  Port=2  Side=Left
  +L3 : PMIOPort  Port=3  Side=Left
  L : PMIOPort  Port=4  Side=Right
  N : PMIOPort  Port=5  Side=Right
  V+ : PMIOPort  Port=6  Side=Right
  V- : PMIOPort  Port=7  Side=Right
  connections:
  +L3/RConn1 -- V+/RConn1
  Electrical Reference3/LConn1 -- V-/RConn1
  L/RConn1 -- +L1/RConn1
  Electrical Reference1/LConn1 -- N/RConn1

== system NHR9410Model96k_2020b/NHR 9410 Mode 9 (Two AC//One DC) Fixture ==
  note: Channel neutral
  Electrical Reference1 : fl_lib/Electrical/Electrical Elements/Electrical Reference
  Electrical Reference2 : fl_lib/Electrical/Electrical Elements/Electrical Reference
  Electrical Reference3 : fl_lib/Electrical/Electrical Elements/Electrical Reference
  +L1 : PMIOPort  Side=Left
  +L2 : PMIOPort  Port=2  Side=Left
  +L3 : PMIOPort  Port=3  Side=Left
  L1 : PMIOPort  Port=4  Side=Right
  N1 : PMIOPort  Port=5  Side=Right
  L2 : PMIOPort  Port=6  Side=Right
  N2 : PMIOPort  Port=7  Side=Right
  V+ : PMIOPort  Port=8  Side=Right
  V- : PMIOPort  Port=9  Side=Right
  connections:
  +L3/RConn1 -- V+/RConn1
  +L2/RConn1 -- L2/RConn1
  Electrical Reference3/LConn1 -- V-/RConn1
  Electrical Reference2/LConn1 -- N2/RConn1
  L1/RConn1 -- +L1/RConn1
  Electrical Reference1/LConn1 -- N1/RConn1

== system NHR9410Model96k_2020b/NHR 9410 Safety Settings ==
  NHR_out : Inport
  Demux : Demux  Outputs=10
  Mux : Mux  Inputs=3
  Mux1 : Mux  Inputs=3
  Safety Ch-1 : Subsystem
  Safety Ch-2 : Subsystem
  Safety Ch-3 : Subsystem
  safety_param ch-1 : Subsystem
  safety_param ch-2 : Subsystem
  safety_param ch-3 : Subsystem
  2Display : Outport  VectorParamsAs1DForOutWhenUnconnected=off
  Trip : Outport  Port=2  VectorParamsAs1DForOutWhenUnconnected=off
  wires:
  NHR_out/1 -> Demux/1
  Safety Ch-2/1(ch-2 trip) -> Mux/2
  Safety Ch-1/1(ch-1 trip) -> Mux/1
  Safety Ch-3/1(ch-3 trip) -> Mux/3
  Mux/1 -> Trip/1
  safety_param ch-1/1(ch-1) -> Safety Ch-1/1(ch-1 out)
  safety_param ch-3/1(ch-3) -> Safety Ch-3/1(ch-3 out)
  safety_param ch-2/1(ch-2) -> Safety Ch-2/1(ch-2 out)
  Demux/1 -> safety_param ch-1/1(P)
  Demux/2 -> safety_param ch-1/2(V)
  Demux/3 -> safety_param ch-1/3(I)
  Demux/4 -> safety_param ch-2/1(P)
  Demux/5 -> safety_param ch-2/2(V)
  Demux/6 -> safety_param ch-2/3(I)
  Demux/7 -> safety_param ch-3/1(P)
  Demux/8 -> safety_param ch-3/2(V)
  Demux/9 -> safety_param ch-3/3(I)
  Demux/10 -> safety_param ch-1/4(hw_mode), safety_param ch-2/4(hw_mode), safety_param ch-3/4(hw_mode)
  safety_param ch-1/2(peak_ctrl) -> Safety Ch-1/2(peak_ctrl)
  safety_param ch-2/2(peak_ctrl) -> Safety Ch-2/2(peak_ctrl)
  safety_param ch-3/2(peak_ctrl) -> Safety Ch-3/2(peak_ctrl)
  Mux1/1 -> 2Display/1
  Safety Ch-1/2(ch-1 trip_all) -> Mux1/1
  Safety Ch-3/2(ch-3 trip_all) -> Mux1/3
  Safety Ch-2/2(ch-2 trip_all) -> Mux1/2

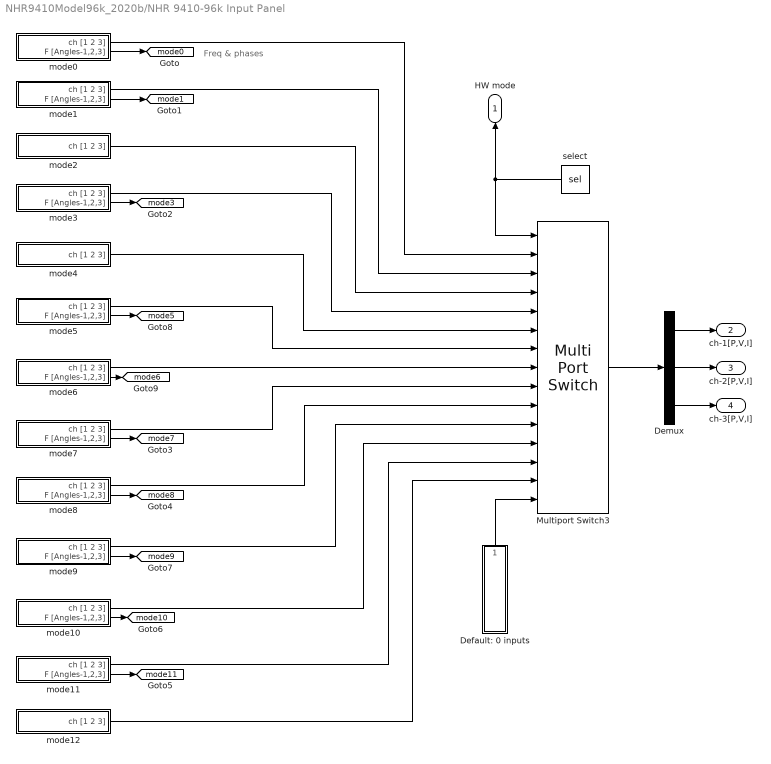
== system NHR9410Model96k_2020b/NHR 9410-96k Input Panel ==
  note: Freq & phases
  Default: 0 inputs : Subsystem
  Demux : Demux  Outputs=3
  Multiport Switch3 : MultiPortSwitch  DataPortOrder=Specify indices  Inputs=13  DataPortIndices={0,1,2,3,4,5,6,7,8,9,10,11,12}  DataPortForDefault=Additional data port  DiagnosticForDefault=None
  mode0 : Subsystem
  mode1 : Subsystem
  mode10 : Subsystem
  mode11 : Subsystem
  mode12 : Subsystem
  mode2 : Subsystem
  mode3 : Subsystem
  mode4 : Subsystem
  mode5 : Subsystem
  mode6 : Subsystem
  mode7 : Subsystem
  mode8 : Subsystem
  mode9 : Subsystem
  select : Constant  Value=sel
  HW mode : Outport  VectorParamsAs1DForOutWhenUnconnected=off
  ch-1[P,V,I] : Outport  Port=2  VectorParamsAs1DForOutWhenUnconnected=off
  ch-2[P,V,I] : Outport  Port=3  VectorParamsAs1DForOutWhenUnconnected=off
  ch-3[P,V,I] : Outport  Port=4  VectorParamsAs1DForOutWhenUnconnected=off
  tag scope: mode0=global, mode10=global, mode11=global, mode1=global, mode3=global, mode5=global, mode6=global, mode7=global, mode8=global, mode9=global
  wires:
  Demux/3 -> ch-3[P,V,I]/1
  Demux/2 -> ch-2[P,V,I]/1
  Demux/1 -> ch-1[P,V,I]/1
  Default: 0 inputs/1(ch [1 2 3]) -> Multiport Switch3/15
  mode0/1(ch [1 2 3]) -> Multiport Switch3/2
  select/1 -> Multiport Switch3/1, HW mode/1
  mode4/1(ch [1 2 3]) -> Multiport Switch3/6
  mode0/2(F [Angles-1,2,3]) -> [mode0]
  mode2/1(ch [1 2 3]) -> Multiport Switch3/4
  mode12/1(ch [1 2 3]) -> Multiport Switch3/14
  mode1/2(F [Angles-1,2,3]) -> [mode1]
  mode1/1(ch [1 2 3]) -> Multiport Switch3/3
  mode3/2(F [Angles-1,2,3]) -> [mode3]
  mode3/1(ch [1 2 3]) -> Multiport Switch3/5
  mode7/1(ch [1 2 3]) -> Multiport Switch3/9
  mode7/2(F [Angles-1,2,3]) -> [mode7]
  mode8/1(ch [1 2 3]) -> Multiport Switch3/10
  mode8/2(F [Angles-1,2,3]) -> [mode8]
  mode11/1(ch [1 2 3]) -> Multiport Switch3/13
  mode11/2(F [Angles-1,2,3]) -> [mode11]
  mode10/1(ch [1 2 3]) -> Multiport Switch3/12
  mode10/2(F [Angles-1,2,3]) -> [mode10]
  mode9/2(F [Angles-1,2,3]) -> [mode9]
  mode9/1(ch [1 2 3]) -> Multiport Switch3/11
  mode5/1(ch [1 2 3]) -> Multiport Switch3/7
  mode5/2(F [Angles-1,2,3]) -> [mode5]
  mode6/1(ch [1 2 3]) -> Multiport Switch3/8
  mode6/2(F [Angles-1,2,3]) -> [mode6]
  Multiport Switch3/1 -> Demux/1

== system NHR9410Model96k_2020b/NHR 9410/Chanel-1 ==
  satefy_trip : Inport
  HW Mode Selection : Inport  Port=2
  Ch-1 input [P V I] : Inport  Port=3
  Chanel-1 Control : Subsystem
  Constant : Constant  Value=p_switch
  Constant4 : Constant  Value=0.1
  Current Sensor : fl_lib/Electrical/Electrical Sensors/Current Sensor
  Logical Operator1 : Logic  AllPortsSameDT=off  OutDataTypeStr=boolean
  Logical Operator2 : Logic  Operator=NOT  AllPortsSameDT=off  OutDataTypeStr=boolean
  NHR 9410 : fl_lib/Electrical/Electrical Sources/Controlled Voltage Source
  PS Constant : fl_lib/Physical Signals/Sources/PS Constant  constant=0
  PS Product1 : fl_lib/Physical Signals/Functions/PS Product
  PS-Simulink Converter1 : nesl_utility/PS-Simulink Converter  PhysicalDomain=network_engine_domain  SubClassName=ps_output  LeftPortType=input  RightPortType=output  PseudoPeriodic=off  Frequencies=[]  Unit=inherit  AffineConversion=off
  PS-Simulink Converter2 : nesl_utility/PS-Simulink Converter  PhysicalDomain=network_engine_domain  SubClassName=ps_output  LeftPortType=input  RightPortType=output  PseudoPeriodic=off  Frequencies=[]  Unit=1  AffineConversion=off
  PS-Simulink Converter4 : nesl_utility/PS-Simulink Converter  PhysicalDomain=network_engine_domain  SubClassName=ps_output  LeftPortType=input  RightPortType=output  PseudoPeriodic=off  Frequencies=[]  Unit=1  AffineConversion=off
  Series Resistor : fl_lib/Electrical/Electrical Elements/Variable Resistor  Rmin=0.0001 Ohm  i_specify=off  i_priority=None  i=0 A  i_nominal_specify=off  i_nominal_unit=A  i_nominal_value=1  v_specify=off  v_priority=None  v=0 V  v_nominal_specify=off  v_nominal_unit=V  v_nominal_value=1
  Simulink-PS Converter : nesl_utility/Simulink-PS Converter  PhysicalDomain=network_engine_domain  SubClassName=ps_input  LeftPortType=input  RightPortType=output  PseudoPeriodic=off  Frequencies=[]  NoiseDistribution=none  NoiseParameters=[]  Unit=1  AffineConversion=off  FilteringAndDerivatives=filter  SimscapeFilterOrder=1  InputFilterTimeConstant=0.001  UdotUserProvided=0
  Switch : Switch  Criteria=u2 > Threshold  ZeroCross=off
  Voltage Sensor1 : fl_lib/Electrical/Electrical Sensors/Voltage Sensor
  + : PMIOPort  Tag=PMCPort  Side=Left
  - : PMIOPort  Tag=PMCPort  Port=2  Side=Left
  Pout : Outport  VectorParamsAs1DForOutWhenUnconnected=off
  Vout : Outport  Port=2  VectorParamsAs1DForOutWhenUnconnected=off
  Iout : Outport  Port=3  VectorParamsAs1DForOutWhenUnconnected=off
  wires:
  Constant/1 -> Logical Operator1/1
  satefy_trip/1 -> Logical Operator2/1
  Logical Operator2/1 -> Logical Operator1/2
  Switch/1 -> Simulink-PS Converter/1
  Chanel-1 Control/1(Vin) -> Switch/1
  Constant4/1 -> Switch/3
  Logical Operator1/1 -> Switch/2
  PS-Simulink Converter2/1 -> Iout/1, Chanel-1 Control/3(Iout)
  PS-Simulink Converter4/1 -> Vout/1, Chanel-1 Control/2(Vout)
  PS-Simulink Converter1/1 -> Pout/1, Chanel-1 Control/1(Pout)
  HW Mode Selection/1 -> Chanel-1 Control/5(HW mode selection)
  Ch-1 input [P V I]/1 -> Chanel-1 Control/4(Ch-1 input [P V I])
  connections:
  Current Sensor/LConn1 -- Series Resistor/RConn1
  PS Constant/RConn1 -- Series Resistor/LConn1
  PS Product1/RConn1 -- PS-Simulink Converter1/LConn1
  Series Resistor/LConn2 -- NHR 9410/LConn1
  Simulink-PS Converter/RConn1 -- NHR 9410/RConn1
  Voltage Sensor1/LConn1 -- +/RConn1 -- Current Sensor/RConn2
  PS-Simulink Converter2/LConn1 -- PS Product1/LConn1 -- Current Sensor/RConn1
  NHR 9410/RConn2 -- -/RConn1 -- Voltage Sensor1/RConn2
  Voltage Sensor1/RConn1 -- PS Product1/LConn2 -- PS-Simulink Converter4/LConn1

== system NHR9410Model96k_2020b/NHR 9410/Chanel-2 ==
  satefy_trip : Inport
  HW Mode Selection : Inport  Port=2
  Ch-2 input [P V I] : Inport  Port=3
  Chanel-2 Control1 : Subsystem
  Constant : Constant  Value=p_switch
  Constant4 : Constant  Value=0.1
  Current Sensor : fl_lib/Electrical/Electrical Sensors/Current Sensor
  Logical Operator1 : Logic  AllPortsSameDT=off  OutDataTypeStr=boolean
  Logical Operator2 : Logic  Operator=NOT  AllPortsSameDT=off  OutDataTypeStr=boolean
  NHR 9410 : fl_lib/Electrical/Electrical Sources/Controlled Voltage Source
  PS Constant : fl_lib/Physical Signals/Sources/PS Constant  constant=0
  PS Product1 : fl_lib/Physical Signals/Functions/PS Product
  PS-Simulink Converter1 : nesl_utility/PS-Simulink Converter  PhysicalDomain=network_engine_domain  SubClassName=ps_output  LeftPortType=input  RightPortType=output  PseudoPeriodic=off  Frequencies=[]  Unit=inherit  AffineConversion=off
  PS-Simulink Converter2 : nesl_utility/PS-Simulink Converter  PhysicalDomain=network_engine_domain  SubClassName=ps_output  LeftPortType=input  RightPortType=output  PseudoPeriodic=off  Frequencies=[]  Unit=1  AffineConversion=off
  PS-Simulink Converter4 : nesl_utility/PS-Simulink Converter  PhysicalDomain=network_engine_domain  SubClassName=ps_output  LeftPortType=input  RightPortType=output  PseudoPeriodic=off  Frequencies=[]  Unit=1  AffineConversion=off
  Series Resistor : fl_lib/Electrical/Electrical Elements/Variable Resistor  Rmin=0.0001 Ohm  i_specify=off  i_priority=None  i=0 A  i_nominal_specify=off  i_nominal_unit=A  i_nominal_value=1  v_specify=off  v_priority=None  v=0 V  v_nominal_specify=off  v_nominal_unit=V  v_nominal_value=1
  Simulink-PS Converter : nesl_utility/Simulink-PS Converter  PhysicalDomain=network_engine_domain  SubClassName=ps_input  LeftPortType=input  RightPortType=output  PseudoPeriodic=off  Frequencies=[]  NoiseDistribution=none  NoiseParameters=[]  Unit=1  AffineConversion=off  FilteringAndDerivatives=filter  SimscapeFilterOrder=1  InputFilterTimeConstant=0.001  UdotUserProvided=0
  Switch : Switch  Criteria=u2 > Threshold  ZeroCross=off
  Voltage Sensor1 : fl_lib/Electrical/Electrical Sensors/Voltage Sensor
  + : PMIOPort  Tag=PMCPort  Side=Left
  - : PMIOPort  Tag=PMCPort  Port=2  Side=Left
  Pout : Outport  VectorParamsAs1DForOutWhenUnconnected=off
  Vout : Outport  Port=2  VectorParamsAs1DForOutWhenUnconnected=off
  Iout : Outport  Port=3  VectorParamsAs1DForOutWhenUnconnected=off
  wires:
  Ch-2 input [P V I]/1 -> Chanel-2 Control1/4(Ch-2 input [P V I])
  HW Mode Selection/1 -> Chanel-2 Control1/5(HW mode selection)
  PS-Simulink Converter1/1 -> Chanel-2 Control1/1(Pout), Pout/1
  PS-Simulink Converter4/1 -> Chanel-2 Control1/2(Vout), Vout/1
  PS-Simulink Converter2/1 -> Chanel-2 Control1/3(Iout), Iout/1
  Logical Operator1/1 -> Switch/2
  Constant4/1 -> Switch/3
  Chanel-2 Control1/1(Vin) -> Switch/1
  Switch/1 -> Simulink-PS Converter/1
  Logical Operator2/1 -> Logical Operator1/2
  satefy_trip/1 -> Logical Operator2/1
  Constant/1 -> Logical Operator1/1
  connections:
  PS-Simulink Converter4/LConn1 -- PS Product1/LConn2 -- Voltage Sensor1/RConn1
  Voltage Sensor1/RConn2 -- -/RConn1 -- NHR 9410/RConn2
  Current Sensor/RConn1 -- PS Product1/LConn1 -- PS-Simulink Converter2/LConn1
  Current Sensor/RConn2 -- +/RConn1 -- Voltage Sensor1/LConn1
  Simulink-PS Converter/RConn1 -- NHR 9410/RConn1
  Series Resistor/LConn2 -- NHR 9410/LConn1
  PS Product1/RConn1 -- PS-Simulink Converter1/LConn1
  PS Constant/RConn1 -- Series Resistor/LConn1
  Current Sensor/LConn1 -- Series Resistor/RConn1
